simulink library "monroe_library"  (R2012b)
settings: Solver=ode45  StartTime=0.0  StopTime=10.0  RelTol=1e-3
values from neighbouring files (symbols this model uses):
  input_bit_width = ', num2str(input_bit_width))    [fft_direct_draw.m]
undefined symbols (not defined in the file or in its folder): gcbh, xlBlockLoadCallback
libraries: xbsIndex_r4 x1880, monroe_library x159, casper_library x13, xps_library x1
(part 1 of 43)
settings Model: Creator=monroe  LastModifiedBy=root

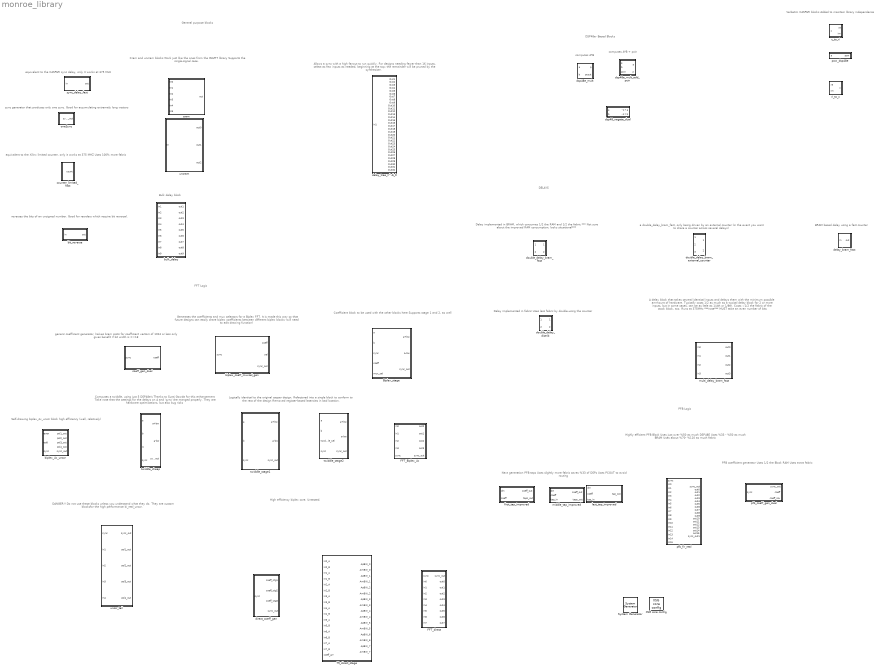
== system monroe_library ==
  note: computes A*B + pcin
  note: equivalent to the CASPER sync delay,
      | only it works at 375 MHz
  note: equivalent to the Xilinx
      | limited counter, only it works at 375 MHZ
      | Uses 100% more fabric
  note: Computes a twiddle, using just 5 DSP48e's
      | Thanks to Suraj Gowda for this enhancement
      | Take note that the settings for the delays on A and 'sync' are manged properly.
      | They are hardware optimizations, but also bug risks
  note: BRAM based delay using a fast counter
  note: sync generator that produces only one sync.
      | Good for accumulating extremely long vectors
  note: computes A*B
  note: Delay implemented in BRAM, which consumes
      | 1/2 the RAM and 1/2 the fabric
      |
      | *** Not sure about the improved RAM consumption; looks situational***
  note: Delay implemented in fabric
      | Uses less fabric by double-using the counter
  note: Next generation PFB taps
      |
      | Uses slightly more fabric
      | saves %33 of DSPs
      | Uses PCOUT to avoid routing
  note: PFB coefficient generator
      | Uses 1/2 the Block RAM
      | Uses extra fabric
  note: Highly efficient PFB Block
      | Uses just over %50 as much DSP48E
      | Uses %33 - %50 as much BRAM
      | Uses about %70- %110 as much fabric
  note: Logically identical to the original casper design.
      | Refactored into a single block to conform to the rest of the design
      | Removed register-based latencies in bad location.
  note: Allows a sync with a high fanout to run quickly.
      |   For designs needing fewer than 16 inputs, select as few inputs as needed, beginning at the top;
      | the remainder will be pruned by the synthesizer.
  note: a double_delay_bram_fast, only being driven by an external counter
      | (in the event you want to share a counter across several delays)
  note: generic coefficient generator,  halves bram costs for coefficient vectors of  1024 or less
      | only gives benefit if bit width is =<18
  note: Cram and uncram blocks
      | Work just like the ones from the GAVRT library
      | Supports the single-signal case.
  note: Generates the coefficients and mux selectors for a Biplex FFT.
      | It is made this way so that future designs can easily share biplex coefficients
      | between different biplex blocks (will need to edit drawing function)
  note: A delay block that takes several identical inputs and
      | delays them with the minimum possible ammount of hardware.
      | Typically costs 1/2 as much as a typical delay block for 2 or more inputs,
      | but in some cases, can be as little as 1/4th or 1/8th.
      | Costs ~1/2 the fabric of the stock block, too.
      | Runs at 375MHz
      |
      | ***note***  MUST take an even number of bits
  note: Verbatim CASPER blocks
      | Added to maintain library independence
  note: DELAYS
  note: PFB Logic
  note: FFT Logic
  note: General purpose blocks
  note: DSP48e- Based Blocks
  note: reverses the bits of an unsigned number.
      | Good for reorders which require bit reversal.
  note: DANGER!!
      | Do not use these blocks unless you understand what they do.
      | They are custom blocksfor the high performance bi_real_unscr.
  note: Coefficient block to be used with the other blocks here
      | Supports stage 1 and 2, as well
  note: Self-drawing biplex_4x_unscr block
      | high efficiency (well, relatively)
  note: High efficiency biplex core.
      | Untested.
  note: Bulk delay block
  " System Generator" : xbsIndex_r4/ System Generator  Tag=genX  xilinxfamily=virtex5  part=xc5vsx95t  speed=-1  package=ff1136  synthesis_tool=XST  clock_wrapper=Clock Enables  directory=./spec_2pol_4kw_6tap_pfb/sysgen  proj_type=Project Navigator  Synth_file=XST Defaults  Impl_file=ISE Defaults  testbench=off  simulink_period=1  sysclk_period=2.6667  dcm_input_clock_period=100  incr_netlist=off  trim_vbits=Everywhere in SubSystem  dbl_ovrd=According to Block Masks  core_generation=According to Block Masks  run_coregen=off  deprecated_control=off  eval_field=0  block_type=sysgen
      settings: block_version=11.4
  Biplex_stage : Subsystem  mask{FFTSize=10, FFTStage=3, input_bit_width=18, coeff_bit_width=18, output_bit_width=18, delays_bram=0, bram_latency=2, shift=0, delay_arr=[0,1,0]}
      mask prompts: FFTSize "FFT Size"; FFTStage "FFT Stage"; input_bit_width "Input Bit Width"; coeff_bit_width "Coefficient Bit Width"; output_bit_width "Output Bit Width"; delays_bram "Delays in BRAM"; bram_latency "BRAM latency"; shift "Downshift in this stage? (0 or 1)"; delay_arr "In-Stage Delay Array"
      mask init:
      | config.source=str2func('biplex_stage_n_draw');
      | config.toplevel=gcb;
      | config.debug=0;
      | config.depend={'biplex_stage_n_draw.m'};
      | xBlock(config,{FFTSize, FFTStage, input_bit_width, coeff_bit_width, output_bit_width, delays_bram, bram_latency, shift, delay_arr});
  FFT_Biplex_4x : Subsystem  mask{FFTSize=10, coeff_bit_width=18, input_bit_width=18, output_bit_width=18, inter_stage_bit_width=18, shift_arr=1, mux_latency_arr=0, max_distro_size_coeff=4, max_distro_size_delay=3, register_coeffs=off, stage_pre_delay=off, stage_mid_delay=off, stage_post_delay=off, bram_latency_fft=off, bram_latency_unscr=off, unscr_din_latency=off}
      mask prompts: FFTSize "FFT Size (2^?) points"; coeff_bit_width "Coefficient Bit Width"; input_bit_width "Input Bit Width"; output_bit_width "Output Bit Width"; inter_stage_bit_width "Inter-Stage Bit Widths"; shift_arr "Shift after n-th stage? (array of FFTSize elements, each a 0 or 1)"; mux_latency_arr "Mux Latency Array"; max_distro_size_coeff "When to start putting Coefficients in BRAM (after 2^? elements)"; max_distro_size_delay "When to start putting Delays in BRAM (after 2^? latency)"; register_coeffs "Register Coefficients?"; stage_pre_delay "Stage Pre-delay? (0 or 1)"; stage_mid_delay "Stage Mid-Delay? (0 or 1)"; stage_post_delay "Stage Post-Delay? (0 or 1)"; bram_latency_fft "Register Bram outputs? (FFT)"; bram_latency_unscr "Register Bram outputs? (Unscrambler)"; unscr_din_latency "Register Unscrambler Reorder inputs?"
      mask init:
      | config.source=str2func('fft_biplex_4x_draw');
      | config.toplevel=gcb;
      | config.debug=0;
      | config.depend={'fft_biplex_4x_draw.m'};
      | xBlock(config,{FFTSize,coeff_bit_width,input_bit_width,output_bit_width,inter_stage_bit_width,shift_arr,max_distro_size_coeff,max_distro_size_delay,register_coeffs,stage_pre_delay,stage_mid_delay,stage_post_delay,mux_latency_arr,bram_latency_fft+2,bram_latency_unscr+2,unscr_din_latency});
  FFT_direct : Subsystem  mask{FFTSize=3, larger_fft_size=9, input_bit_width=18, coeff_bit_width=18, inter_stage_bit_width=18, output_bit_width=18, register_coeffs=on, delay_input=on, delay_output=off, sync_tree_input=off, optional_delay_arr=1, coeff_group_arr_in=[], coeff_stage_step_arr=0, shift_arr=1}
      mask prompts: FFTSize "FFT Size"; larger_fft_size "Larger FFT Size"; input_bit_width "Input Bit Width (no more than 24)"; coeff_bit_width "Coeff Bit Width (Array, FFT Size long; max 18)"; inter_stage_bit_width "Inter-Stage Bit Width (Array, FFT Size -1 long, max 24)"; output_bit_width "Output Bit Width (positive integer)"; register_coeffs "Register Coefficients?"; delay_input "Delay Input?"; delay_output "Delay Output?"; sync_tree_input "Add Sync Tree to Input?"; optional_delay_arr "Optional Delays (array, FFT Size-1 long)"; coeff_group_arr_in "Coefficient Grouping Array (read documentation or use empty array  []   )"; coeff_stage_step_arr "Coefficient Stage Step Size (array of FFT Size, non-negative integers)"; shift_arr "Stage Shift Array (array of FFT Size, non-negative integers; recomend ones(1,FFTSize))"
      mask init:
      | config.source=str2func('fft_direct_draw');
      | config.toplevel=gcb;
      | config.debug=0;
      | config.depend={'fft_direct_draw.m'};
      | xBlock(config,{FFTSize,larger_fft_size,input_bit_width,coeff_bit_width,inter_stage_bit_width,output_bit_width,register_coeffs,delay_input,delay_output,sync_tree_input,optional_delay_arr,coeff_group_arr_in,coeff_stage_step_arr,shift_arr});
  XSG core config : xps_library/XSG core config  Tag=xps:xsg  hw_sys=ROACH:sx95t  clk_src=adc0_clk  ROACH_clk_src=adc0_clk  ROACH2_clk_src=adc0_clk  clk_rate=375  sample_period=1  synthesis_tool=XST
  biplex_4x_unscr : Subsystem  mask{FFTSize=9, bram_latency=3, input_bit_width=18, reorder_din_latency=1}
      mask prompts: FFTSize "Size of FFT (2^?):"; bram_latency "BRAM Latency"; input_bit_width "Input Bit Width"; reorder_din_latency "Reorder Data In Latency"
      mask init:
      | config.source=str2func('biplex_4x_unscr_draw');
      | config.toplevel=gcb;
      | config.debug=0;
      | config.depend={'biplex_4x_unscr_draw.m'};
      | xBlock(config,{FFTSize, bram_latency, input_bit_width, reorder_din_latency});
  biplex_coeff_muxsel_gen : Subsystem  mask{FFTSize=4, bit_width=18*ones(1,2), register_coeffs=0, max_distro_size=4, optional_delay_arr=[[1,1,1]; [1,1,1];  [1,1,1];  [1,1,1]], stage_delay_arr=[3,6,6,6]}
      mask prompts: FFTSize "FFT Size"; bit_width "Coefficient Bit Width"; register_coeffs "Register Coeffs?"; max_distro_size "Maximum number of coeffs to put in distributed memory? (2^? points)"; optional_delay_arr "In-Stage Delay Array"; stage_delay_arr "Mandatory Stage Delay Array"
      mask init:
      | config.source=str2func('biplex_coeff_muxsel_gen_draw');
      | config.toplevel=gcb;
      | config.debug=0;
      | config.depend={'biplex_coeff_muxsel_gen_draw.m'};
      | xBlock(config,{FFTSize, bit_width, register_coeffs, max_distro_size, optional_delay_arr, stage_delay_arr});
  bit_reverse : Subsystem  mask{nBits=5}
      mask prompts: nBits "# bits?"
      mask init:
      | config.source=str2func('bit_reverse_draw');
      | config.toplevel=gcb;
      | config.debug=0;
      | config.depend={'bit_reverse_draw.m'};
      | xBlock(config,{nBits,1});
  bulk_delay : Subsystem  mask{numInputs=9, delay_arr=5}
      mask prompts: numInputs "# Inputs?"; delay_arr "Delays (integer or array of #inputs elements)"
      mask init:
      | config.source=str2func('bulk_delay_draw');
      | config.toplevel=gcb;
      | config.debug=0;
      | config.depend={'bulk_delay_draw.m'};
      | xBlock(config,{numInputs,delay_arr});
  c_to_ri : Subsystem  AncestorBlock=casper_library/Misc/c_to_ri  mask(c_to_ri){n_bits=8, bin_pt=7}
      mask prompts: n_bits "Bit Width"; bin_pt "Binary Point"
      mask help:
      | Outputs real and imaginary components of a complex input.
      | Useful for simplifying interconnects.
      | See also: Real-Imag to Complex (ri_to_c)
      mask init:
      | annotation=sprintf('%d_%d r/i',n_bits,bin_pt);
      | set_param(gcb,'AttributesFormatString',annotation);
      settings: AttributesFormatString=8_7 r/i
      mask Help: eval('xlWeb(''http://casper.berkeley.edu/wiki/C_to_ri'')')
  coeff_gen_dual : Subsystem  mask{coeff=(1:128)/128, memory_type=Block RAM, bit_width=18, register_output=0, step_rate=0}
      mask prompts: coeff "Coefficients"; memory_type "Memory Type"; bit_width "Bit Width"; register_output "Register Output? (does not affect latency)"; step_rate "Step Rate"
      mask init:
      | config.source=str2func('coeff_gen_dual_draw');
      | config.toplevel=gcb;
      | config.debug=0;
      | config.depend={'coeff_gen_dual_draw.m'};
      | xBlock(config,{coeff, memory_type, bit_width, step_rate, register_output});
      mask TypeOptions memory_type: Block RAM | Distributed memory
  counter_limited_fast : Subsystem  mask{bit_width=8, count_to=250, register_output=0, cheap_counter=0}
      mask prompts: bit_width "Bit Width"; count_to "Max Counter Value"; register_output "Register Output? (0 or 1)"; cheap_counter "Use Cheap Counter Instead?"
  cram : Subsystem  mask{numInputs=6}
      mask prompts: numInputs "# Inputs"
      mask init:
      | config.source=str2func('cram_draw');
      | config.toplevel=gcb;
      | config.debug=0;
      | config.depend={'cram_draw.m'};
      | xBlock(config,{numInputs});
  delay_bram_fast : Subsystem  AncestorBlock=monroe_library/tap1/delay_bram  mask{delay_len=1024, bram_latency=2, memory_type=Block RAM, register_counter=0}
      mask prompts: delay_len "Delay Length"; bram_latency "Bram Latency"; memory_type "Memory Type"; register_counter "Register internal counter? (0 or 1)"
      mask TypeOptions memory_type: Block RAM | Distributed Memory
  delay_tree_z^-6_0 : Subsystem
  direct_coeff_gen : Subsystem  mask{fft_size=3, larger_fft_size=13, bit_width=18*ones(1,3), register_coeffs=0, delay_input=1, sync_tree_input=0, optional_delay_arr=[1,1,1], coeff_group_arr=[], coeff_stage_step_arr=zeros(1,3)}
      mask prompts: fft_size "FFT Size"; larger_fft_size "Larger FFT Size"; bit_width "Coeff bit width"; register_coeffs "Register Coefficients"; delay_input "Register Inputs"; sync_tree_input "Attach Sync-Tree to input (0 or 1)"; optional_delay_arr "Optional Delay Array"; coeff_group_arr "Coeff Group Array"; coeff_stage_step_arr "Coeff Stage Step Array"
      mask init:
      | config.source=str2func('direct_coeff_gen_draw');
      | config.toplevel=gcb;
      | config.debug=0;
      | config.depend={'direct_coeff_gen_draw.m'};
      | xBlock(config,{fft_size, larger_fft_size, bit_width, register_coeffs, delay_input, sync_tree_input, optional_delay_arr, coeff_group_arr, coeff_stage_step_arr});
  double_delay_bram_external_counter : Subsystem  mask{delay_len=1024, bram_latency=2}
      mask prompts: delay_len "Delay Length"; bram_latency "Bram Latency"
  double_delay_bram_fast : Subsystem  mask{delay_len=1024, bram_latency=2, register_counter=0}
      mask prompts: delay_len "Delay Length"; bram_latency "Bram Latency"; register_counter "Register Internal Counter? (0 or 1)"
  double_delay_distrib : Subsystem  mask{delay_len=1024, bram_latency=2}
      mask prompts: delay_len "Delay Length"; bram_latency "Bram Latency"
  dsp48_negate_dual : Subsystem  mask{a_bit_width=input_bit_width, a_bin_pt=input_bit_width-1}
      mask prompts: a_bit_width "bit width"; a_bin_pt "binary point"
  dsp48e_mult : Subsystem  mask{a_bin_pt=17, b_bin_pt=17}
      mask prompts: a_bin_pt "'A' binal point"; b_bin_pt "'B' binal point"
  dsp48e_mult_add_pcin : Subsystem  mask{a_bin_pt=0, b_bin_pt=0}
      mask prompts: a_bin_pt "'A' binal point"; b_bin_pt "'B' binal point"
  fft_direct_stage : Subsystem  mask{FFTSize=4, FFTStage=3, input_bit_width=18, coeff_bit_width=18, output_bit_width=18, shift=1}
      mask prompts: FFTSize "FFT Size"; FFTStage "FFT Stage"; input_bit_width "Input Bit Width"; coeff_bit_width "Coeff Bit Width"; output_bit_width "Output Bit Width"; shift "Downshift stage output?"
      mask init:
      | config.source=str2func('fft_direct_stage_draw');
      | config.toplevel=gcb;
      | config.debug=0;
      | config.depend={'fft_direct_stage_draw.m'};
      | xBlock(config,{FFTSize, FFTStage, input_bit_width, coeff_bit_width, output_bit_width, shift});
  first_tap_improved : Subsystem  AncestorBlock=casper_library/PFBs/tap_real  mask{data_bin_pt=17, coeff_bit_width=18}
      mask prompts: data_bin_pt "Data Binal Point"; coeff_bit_width "Coefficient Bit Width (max 25)"
  last_tap_improved : Subsystem  AncestorBlock=casper_library/PFBs/last_tap_real  mask{data_bin_pt=17, coeff_bin_pt=17, stage_num=6}
      mask prompts: data_bin_pt "Data Binal Point"; coeff_bin_pt "Coeficient Binal Point"; stage_num "Stage Number"
  middle_tap_improved : Subsystem  mask{data_bin_pt=17, coeff_bit_width=18, stage_num=2}
      mask prompts: data_bin_pt "Data Binal Point"; coeff_bit_width "Coefficient Bit Width (max 25)"; stage_num "Stage Number"
  multi_delay_bram_fast : Subsystem  mask{numSignals=4, delay_len=1024, bitWidth=18, binPt=17, signalType=Signed, bram_latency=2, register_counter=0}
      mask prompts: numSignals "# signals"; delay_len "Delay Length"; bitWidth "Bit Width"; binPt "Binal Point"; signalType "Signal Type"; bram_latency "Bram Latency"; register_counter "Register internal counter? (0 or 1)"
      mask init:
      | config.source=str2func('multi_delay_bram_fast_draw');
      | config.toplevel=gcb;
      | config.debug=0;
      | config.depend={'multi_delay_bram_fast_draw.m','cram_draw.m', 'uncram_draw.m'};
      | xBlock(config,{numSignals, delay_len, bitWidth, binPt, signalType, bram_latency,register_counter});
      mask TypeOptions signalType: Signed | Unsigned
  oneSync : Subsystem
  pfb_coeff_gen_dual : Subsystem  mask(pfb_coeff_gen_dual){pfb_size=14, n_sim_inputs=4, n_taps=4, input_num=4, n_bits=18, window_fn=hamming, mem_type=Block RAM, bram_latency=3, bin_width=1}
      mask prompts: pfb_size "PFB Size (2^?)"; n_sim_inputs "# Simultaneous Inputs (2^?)"; n_taps "# Taps"; input_num "Input Number (zero-indexed)"; n_bits "# Coefficient Bits"; window_fn "Window Function"; mem_type "Memory Type"; bram_latency "Bram Latency (reccomend 3)"; bin_width "Channel Width"
      mask init:
      | % wampum=55;
      | % 
      | config.source = str2func('pfb_coeff_gen_dual_draw');
      | config.toplevel=gcb;
      | config.debug=0;
      | config.depend = {'pfb_coeff_gen_dual_draw.m'};
      | 
      | %parameters to pass to drawer
      |     global drawing_parameters;
      |     drawing_parameters.pfb_size=pfb_size;
      |     drawing_parameters.n_sim_inputs=n_sim_inputs;
      |     drawing_parameters.n_taps=n_taps;
      |     drawing_parameters.input_num=input_num;
      |     drawing_parameters.n_bits=n_bits;
      |     drawing_parameters.window_fn=window_fn;
      |     drawing_parameters.mem_type=mem_type;
      |     drawing_parameters.bram_latency=bram_latency;
      |     drawing_parameters.bin_width=bin_width;
      |     drawing_parameters.params_from_struct = 0;
      |     
      | 
      | 
      | xBlock(config, {pfb_size,n_sim_inputs,n_taps,input_num,n_bits,window_fn,mem_type,bram_latency,bin_width})
      | 
      | % %pfb_coeff_gen_dual_draw('pfb_size', pfb_size,'n_sim_inputs',n_sim_inputs,'n_taps',n_taps,'input_num',input_num,'n_bits',n_bits,'window_fn',window_fn,'mem_type',mem_type,'bram_latency',bram_latency,'bin_width',bin_width)
      mask TypeOptions window_fn: bartlett | barthannwin | blackman | blackmanharris | bohamwin | chebwin | flattopwin | gausswin | hamming | hann | kaiser | nuttallwin | parzenwin | rectwin | tukeywin | triang
      mask TypeOptions mem_type: Block RAM | Distributed Memory
  pfb_fir_real : Subsystem  mask(pfb_coeff_gen_dual){pfb_size=14, n_sim_inputs=4, n_taps=4, data_n_bits=18, coeff_n_bits=18, output_bit_width=18, window_fn=hamming, bin_width=1, end_scale_val=1, endDelay=off, cheap_sync=off, autoplace_mode='Attached to both ADC0 and ADC1 (interleaved)', autoplace_optimize=off, bram_latency_coeff=off, bram_latency_delay=off, register_counter=off, pack_delays=on}
      mask prompts: pfb_size "PFB Size (2^?)"; n_sim_inputs "# Simultaneous Inputs (2^?); Max=6"; n_taps "# Taps"; data_n_bits "Input bit Width"; coeff_n_bits "# Coefficient Bits"; output_bit_width "Output bit width"; window_fn "Window Function"; bin_width "Channel Width"; end_scale_val "Downscale at end (2^?)"; endDelay "Delay at end?"; cheap_sync "Use cheap Sync hardware?"; autoplace_mode "Autoplacement Mode?"; autoplace_optimize "Optimize parameters for auto-placement? (settings below here ignored)"; bram_latency_coeff "Regoster Coefficient Brams?"; bram_latency_delay "Register Delay Brams?"; register_counter "Register Delay Counters? (0 or 1)"; pack_delays "Pack delays cross-input?"
      mask init:
      | global drawing_parameters;
      | % drawing_parameters.pfb_size=pfb_size;
      | % drawing_parameters.n_sim_inputs=n_sim_inputs;
      | % drawing_parameters.n_taps=n_taps;
      | % drawing_parameters.data_n_bits=data_n_bits;
      | % drawing_parameters.data_bin_pt=data_bin_pt;
      | % drawing_parameters.coeff_n_bits=coeff_n_bits;
      | % drawing_parameters.coeff_bin_pt=coeff_n_bits-1;
      | % drawing_parameters.window_fn=window_fn;
      | % drawing_parameters.mem_type=mem_type;
      | % drawing_parameters.bram_latency=bram_latency;
      | % drawing_parameters.bin_width=bin_width;
      | % drawing_parameters.end_scale_val=end_scale_val;
      | % drawing_parameters.cheap_sync=cheap_sync;
      | config.source=str2func('pfb_improved_draw');
      | config.toplevel=gcb;
      | config.debug=0;
      | config.depend={'pfb_improved_draw.m','pfb_coeff_gen_dual_draw.m'};
      | xBlock(config,{pfb_size,n_sim_inputs,n_taps,data_n_bits,coeff_n_bits, ...
      |                output_bit_width,window_fn,bram_latency_coeff+2,bram_latency_delay+2,bin_width,end_scale_val,endDelay, cheap_sync,register_counter, pack_delays, autoplace_mode, autoplace_optimize});
      mask TypeOptions window_fn: bartlett | barthannwin | blackman | blackmanharris | bohamwin | chebwin | flattopwin | gausswin | hamming | hann | kaiser | nuttallwin | parzenwin | rectwin | tukeywin | triang
      mask TypeOptions autoplace_mode: 'Attached to ADC0' | 'Attached to ADC1' | 'Attached to both ADC0 and ADC1 (interleaved)'
  pow_dsp48e : Subsystem  AncestorBlock=casper_library/Misc/pow_dsp48e  mask{bit_width=8}
      mask prompts: bit_width "Bit Width"
  ri_to_c : Subsystem  AncestorBlock=casper_library/Misc/ri_to_c  mask(ri_to_c){}
      mask help:
      | Concatenates real and imaginary inputs into a complex output.
      | Useful for simplifying interconnects.
      | See also: Complex to Real-Imag (c_to_ri)
      mask Help: eval('xlWeb(''http://casper.berkeley.edu/wiki/Ri_to_c'')')
  sync_delay_fast : Subsystem  mask{delay_len=1024}
      mask prompts: delay_len "Delay Length"
      mask Display: fprintf('Z^-%d', delay_len)
  twiddle_cheap : Subsystem  AncestorBlock=monroe_library/twiddle_cheap  mask{a_n_bits=18, a_bin_pt=17, b_n_bits=18, b_bin_pt=17, w_n_bits=18, w_bin_pt=17, a_delay=0, apbw_delay=0, out_n_bits=18, downshift_at_end=0}
      mask prompts: a_n_bits "# bits A"; a_bin_pt "A binal point"; b_n_bits "# bits B"; b_bin_pt "B binal point"; w_n_bits "# bits W"; w_bin_pt "W binal point"; a_delay "Delay 'A' in-block? (0 or 1)"; apbw_delay "Delay 'A+BW' in-block? (0 or 1)"; out_n_bits "#bits Out"; downshift_at_end "Downshift at end? (0 or 1)"
  twiddle_stage1 : Subsystem  AncestorBlock=monroe_library/twiddle_stage1  mask(twiddle_pass_through){input_bit_width=18, out_n_bits=0, downshift_at_end=0}
      mask prompts: input_bit_width "Input Bit Width"; out_n_bits "Output Bit Width"; downshift_at_end "Downshift at end"
      mask help:
      | Used in FFT library. Used when coefficients
      | are 2^0 i.e just pass data through without delays
  twiddle_stage2 : Subsystem  AncestorBlock=casper_library/FFTs/Twiddle/twiddle_pass_through  mask(twiddle_pass_through){FFTSize=10, input_bit_width=18, out_n_bits=0, downshift_at_end=0}
      mask prompts: FFTSize "FFT Size"; input_bit_width "Input Bit Width"; out_n_bits "Output  Bit Width"; downshift_at_end "Downshift at end (0 or 1)"
      mask help:
      | Used in FFT library. Used when coefficients
      | are 2^0 i.e just pass data through without delays
  uncram : Subsystem  mask{numInputs=3, bitWidth=18, binPt=17, signalType=Signed}
      mask prompts: numInputs "# Inputs"; bitWidth "Bit Width"; binPt "Binal Point"; signalType "Signal Type"
      mask init:
      | config.source=str2func('uncram_draw');
      | config.toplevel=gcb;
      | config.debug=0;
      | config.depend={'uncram_draw.m'};
      | xBlock(config,{numInputs,bitWidth,binPt,signalType});
      mask TypeOptions signalType: Signed | Unsigned
  unscr_tail : Subsystem  AncestorBlock=monroe_library/unscr_tail  mask{FFTSize=5, input_bit_width=18, bram_latency=2, reorder_din_latency=0}
      mask prompts: FFTSize "FFT Size"; input_bit_width "Input Bit Width"; bram_latency "BRAM Latency"; reorder_din_latency "Reorder DIN Latency"

== system monroe_library/Biplex_stage ==
  a : Inport
  b : Inport  Port=2
  sync : Inport  Port=3
  coeff : Inport  Port=4
  mux_sel : Inport  Port=5
  Mux : xbsIndex_r4/Mux  inputs=2  en=off  latency=0  precision=Full  arith_type="Signed  (2's comp)"  n_bits=8  bin_pt=2  quantization=Truncate  overflow=Wrap  dbl_ovrd=off  block_type=mux
  Mux1 : xbsIndex_r4/Mux  inputs=2  en=off  latency=0  precision=Full  arith_type="Signed  (2's comp)"  n_bits=8  bin_pt=2  quantization=Truncate  overflow=Wrap  dbl_ovrd=off  block_type=mux
  delay_ddbf_1 : xbsIndex_r4/Delay  en=off  latency=128  dbl_ovrd=off  reg_retiming=off  block_type=delay
  delay_ddbf_2 : xbsIndex_r4/Delay  en=off  latency=128  dbl_ovrd=off  reg_retiming=off  block_type=delay
  delay_end : xbsIndex_r4/Delay  en=off  latency=2  dbl_ovrd=off  reg_retiming=off  block_type=delay
  delay_mid : xbsIndex_r4/Delay  en=off  latency=2  dbl_ovrd=off  reg_retiming=off  block_type=delay
  delay_mid1 : xbsIndex_r4/Delay  en=off  latency=1  dbl_ovrd=off  reg_retiming=off  block_type=delay
  sync_delay_fast : monroe_library/sync_delay_fast  SystemSampleTime=-1  delay_len=128
  twiddle_cheap : monroe_library/twiddle_cheap  SystemSampleTime=-1  a_n_bits=18  a_bin_pt=17  b_n_bits=18  b_bin_pt=17  w_n_bits=18  w_bin_pt=17  a_delay=0  apbw_delay=0  out_n_bits=18  downshift_at_end=0
  a+bw : Outport
  a-bw : Outport  Port=2
  sync_out : Outport  Port=3
  wires:
  mux_sel/1 -> Mux1/1, Mux/1
  delay_ddbf_2/1 -> Mux1/3, Mux/2
  a/1 -> Mux1/2, Mux/3
  twiddle_cheap/3 -> sync_out/1
  twiddle_cheap/2 -> a-bw/1
  twiddle_cheap/1 -> delay_end/1
  sync_delay_fast/1 -> twiddle_cheap/4
  coeff/1 -> twiddle_cheap/3
  delay_mid1/1 -> twiddle_cheap/2
  delay_mid/1 -> twiddle_cheap/1
  sync/1 -> sync_delay_fast/1
  b/1 -> delay_ddbf_2/1
  Mux/1 -> delay_mid1/1
  delay_ddbf_1/1 -> delay_mid/1
  delay_end/1 -> a+bw/1
  Mux1/1 -> delay_ddbf_1/1

== system monroe_library/FFT_Biplex_4x ==
  in0 : Inport
  in1 : Inport  Port=2
  in2 : Inport  Port=3
  in3 : Inport  Port=4
  sync : Inport  Port=5
  biplex_4x_unscr : Subsystem
  biplex_muxsel_gen : Subsystem
  coeff_slice10 : xbsIndex_r4/Slice  nbits=36  boolean_output=off  mode=Upper Bit Location + Width  bit1=-252  base1=MSB of Input  bit0=-252  base0=MSB of Input  dbl_ovrd=off  block_type=slice
  coeff_slice3 : xbsIndex_r4/Slice  nbits=36  boolean_output=off  mode=Upper Bit Location + Width  bit1=-0  base1=MSB of Input  bit0=-0  base0=MSB of Input  dbl_ovrd=off  block_type=slice
  coeff_slice4 : xbsIndex_r4/Slice  nbits=36  boolean_output=off  mode=Upper Bit Location + Width  bit1=-36  base1=MSB of Input  bit0=-36  base0=MSB of Input  dbl_ovrd=off  block_type=slice
  coeff_slice5 : xbsIndex_r4/Slice  nbits=36  boolean_output=off  mode=Upper Bit Location + Width  bit1=-72  base1=MSB of Input  bit0=-72  base0=MSB of Input  dbl_ovrd=off  block_type=slice
  coeff_slice6 : xbsIndex_r4/Slice  nbits=36  boolean_output=off  mode=Upper Bit Location + Width  bit1=-108  base1=MSB of Input  bit0=-108  base0=MSB of Input  dbl_ovrd=off  block_type=slice
  coeff_slice7 : xbsIndex_r4/Slice  nbits=36  boolean_output=off  mode=Upper Bit Location + Width  bit1=-144  base1=MSB of Input  bit0=-144  base0=MSB of Input  dbl_ovrd=off  block_type=slice
  coeff_slice8 : xbsIndex_r4/Slice  nbits=36  boolean_output=off  mode=Upper Bit Location + Width  bit1=-180  base1=MSB of Input  bit0=-180  base0=MSB of Input  dbl_ovrd=off  block_type=slice
  coeff_slice9 : xbsIndex_r4/Slice  nbits=36  boolean_output=off  mode=Upper Bit Location + Width  bit1=-216  base1=MSB of Input  bit0=-216  base0=MSB of Input  dbl_ovrd=off  block_type=slice
  cram0 : Subsystem
  cram1 : Subsystem
  sel_slice1 : xbsIndex_r4/Slice  nbits=1  boolean_output=on  mode=Upper Bit Location + Width  bit1=-0  base1=MSB of Input  bit0=-0  base0=MSB of Input  dbl_ovrd=off  block_type=slice
  sel_slice10 : xbsIndex_r4/Slice  nbits=1  boolean_output=on  mode=Upper Bit Location + Width  bit1=-9  base1=MSB of Input  bit0=-9  base0=MSB of Input  dbl_ovrd=off  block_type=slice
  sel_slice2 : xbsIndex_r4/Slice  nbits=1  boolean_output=on  mode=Upper Bit Location + Width  bit1=-1  base1=MSB of Input  bit0=-1  base0=MSB of Input  dbl_ovrd=off  block_type=slice
  sel_slice3 : xbsIndex_r4/Slice  nbits=1  boolean_output=on  mode=Upper Bit Location + Width  bit1=-2  base1=MSB of Input  bit0=-2  base0=MSB of Input  dbl_ovrd=off  block_type=slice
  sel_slice4 : xbsIndex_r4/Slice  nbits=1  boolean_output=on  mode=Upper Bit Location + Width  bit1=-3  base1=MSB of Input  bit0=-3  base0=MSB of Input  dbl_ovrd=off  block_type=slice
  sel_slice5 : xbsIndex_r4/Slice  nbits=1  boolean_output=on  mode=Upper Bit Location + Width  bit1=-4  base1=MSB of Input  bit0=-4  base0=MSB of Input  dbl_ovrd=off  block_type=slice
  sel_slice6 : xbsIndex_r4/Slice  nbits=1  boolean_output=on  mode=Upper Bit Location + Width  bit1=-5  base1=MSB of Input  bit0=-5  base0=MSB of Input  dbl_ovrd=off  block_type=slice
  sel_slice7 : xbsIndex_r4/Slice  nbits=1  boolean_output=on  mode=Upper Bit Location + Width  bit1=-6  base1=MSB of Input  bit0=-6  base0=MSB of Input  dbl_ovrd=off  block_type=slice
  sel_slice8 : xbsIndex_r4/Slice  nbits=1  boolean_output=on  mode=Upper Bit Location + Width  bit1=-7  base1=MSB of Input  bit0=-7  base0=MSB of Input  dbl_ovrd=off  block_type=slice
  sel_slice9 : xbsIndex_r4/Slice  nbits=1  boolean_output=on  mode=Upper Bit Location + Width  bit1=-8  base1=MSB of Input  bit0=-8  base0=MSB of Input  dbl_ovrd=off  block_type=slice
  stage_1 : Subsystem
  stage_10 : Subsystem
  stage_2 : Subsystem
  stage_3 : Subsystem
  stage_4 : Subsystem
  stage_5 : Subsystem
  stage_6 : Subsystem
  stage_7 : Subsystem
  stage_8 : Subsystem
  stage_9 : Subsystem
  out0 : Outport
  out1 : Outport  Port=2
  out2 : Outport  Port=3
  out3 : Outport  Port=4
  sync_out : Outport  Port=5
  wires:
  sync/1 -> stage_1/3(sync), biplex_muxsel_gen/1(sync)
  biplex_muxsel_gen/2(sel) -> sel_slice10/1, sel_slice9/1, sel_slice8/1, sel_slice7/1, sel_slice6/1, sel_slice5/1, sel_slice4/1, sel_slice3/1, sel_slice2/1, sel_slice1/1
  biplex_muxsel_gen/1(coeff) -> coeff_slice10/1, coeff_slice9/1, coeff_slice8/1, coeff_slice7/1, coeff_slice6/1, coeff_slice5/1, coeff_slice4/1, coeff_slice3/1
  biplex_4x_unscr/5(sync_out) -> sync_out/1
  biplex_4x_unscr/4(pol4_out) -> out3/1
  biplex_4x_unscr/3(pol3_out) -> out2/1
  biplex_4x_unscr/2(pol2_out) -> out1/1
  biplex_4x_unscr/1(pol1_out) -> out0/1
  biplex_muxsel_gen/3(sync_out) -> biplex_4x_unscr/3(sync)
  stage_10/2(a-bw) -> biplex_4x_unscr/2(odd)
  stage_10/1(a+bw) -> biplex_4x_unscr/1(even)
  sel_slice10/1 -> stage_10/5(mux_sel)
  coeff_slice10/1 -> stage_10/4(coeff)
  stage_9/3(sync_out) -> stage_10/3(sync)
  stage_9/2(a-bw) -> stage_10/2(b)
  stage_9/1(a+bw) -> stage_10/1(a)
  sel_slice9/1 -> stage_9/5(mux_sel)
  coeff_slice9/1 -> stage_9/4(coeff)
  stage_8/3(sync_out) -> stage_9/3(sync)
  stage_8/2(a-bw) -> stage_9/2(b)
  stage_8/1(a+bw) -> stage_9/1(a)
  sel_slice8/1 -> stage_8/5(mux_sel)
  coeff_slice8/1 -> stage_8/4(coeff)
  stage_7/3(sync_out) -> stage_8/3(sync)
  stage_7/2(a-bw) -> stage_8/2(b)
  stage_7/1(a+bw) -> stage_8/1(a)
  sel_slice7/1 -> stage_7/5(mux_sel)
  coeff_slice7/1 -> stage_7/4(coeff)
  stage_6/3(sync_out) -> stage_7/3(sync)
  stage_6/2(a-bw) -> stage_7/2(b)
  stage_6/1(a+bw) -> stage_7/1(a)
  sel_slice6/1 -> stage_6/5(mux_sel)
  coeff_slice6/1 -> stage_6/4(coeff)
  stage_5/3(sync_out) -> stage_6/3(sync)
  stage_5/2(a-bw) -> stage_6/2(b)
  stage_5/1(a+bw) -> stage_6/1(a)
  sel_slice5/1 -> stage_5/5(mux_sel)
  coeff_slice5/1 -> stage_5/4(coeff)
  stage_4/3(sync_out) -> stage_5/3(sync)
  stage_4/2(a-bw) -> stage_5/2(b)
  stage_4/1(a+bw) -> stage_5/1(a)
  sel_slice4/1 -> stage_4/5(mux_sel)
  coeff_slice4/1 -> stage_4/4(coeff)
  stage_3/3(sync_out) -> stage_4/3(sync)
  stage_3/2(a-bw) -> stage_4/2(b)
  stage_3/1(a+bw) -> stage_4/1(a)
  sel_slice3/1 -> stage_3/5(mux_sel)
  coeff_slice3/1 -> stage_3/4(coeff)
  stage_2/3(sync_out) -> stage_3/3(sync)
  stage_2/2(a-bw) -> stage_3/2(b)
  stage_2/1(a+bw) -> stage_3/1(a)
  sel_slice2/1 -> stage_2/4(mux_sel)
  stage_1/3(sync_out) -> stage_2/3(sync)
  stage_1/2(a-bw) -> stage_2/2(b)
  stage_1/1(a+bw) -> stage_2/1(a)
  sel_slice1/1 -> stage_1/4(mux_sel)
  cram1/1(out) -> stage_1/2(b)
  cram0/1(out) -> stage_1/1(a)
  in3/1 -> cram1/2(in1)
  in2/1 -> cram1/1(in0)
  in1/1 -> cram0/2(in1)
  in0/1 -> cram0/1(in0)

== system monroe_library/FFT_direct ==
  sync : Inport
  in0 : Inport  Port=2
  in1 : Inport  Port=3
  in2 : Inport  Port=4
  in3 : Inport  Port=5
  in4 : Inport  Port=6
  in5 : Inport  Port=7
  in6 : Inport  Port=8
  in7 : Inport  Port=9
  bulk_delay_0_1 : Subsystem
  bulk_delay_1_1 : Subsystem
  bulk_delay_2_1 : Subsystem
  bulk_delay_3_1 : Subsystem
  direct_coeff_gen : Subsystem
  stage_1 : Subsystem
  stage_2 : Subsystem
  stage_3 : Subsystem
  sync_out : Outport
  out0 : Outport  Port=2
  out1 : Outport  Port=3
  out2 : Outport  Port=4
  out3 : Outport  Port=5
  out4 : Outport  Port=6
  out5 : Outport  Port=7
  out6 : Outport  Port=8
  out7 : Outport  Port=9
  wires:
  bulk_delay_3_1/8(out8) -> out7/1
  bulk_delay_3_1/7(out7) -> out6/1
  bulk_delay_3_1/6(out6) -> out5/1
  bulk_delay_3_1/5(out5) -> out4/1
  bulk_delay_3_1/4(out4) -> out3/1
  bulk_delay_3_1/3(out3) -> out2/1
  bulk_delay_3_1/2(out2) -> out1/1
  bulk_delay_3_1/1(out1) -> out0/1
  stage_3/8(AmBW_3) -> bulk_delay_3_1/8(in8)
  stage_3/4(AmBW_1) -> bulk_delay_3_1/7(in7)
  stage_3/6(AmBW_2) -> bulk_delay_3_1/6(in6)
  stage_3/2(AmBW_0) -> bulk_delay_3_1/5(in5)
  stage_3/7(ApBW_3) -> bulk_delay_3_1/4(in4)
  stage_3/3(ApBW_1) -> bulk_delay_3_1/3(in3)
  stage_3/5(ApBW_2) -> bulk_delay_3_1/2(in2)
  stage_3/1(ApBW_0) -> bulk_delay_3_1/1(in1)
  direct_coeff_gen/3(coeff_stg3) -> stage_3/9(coeff_arr)
  bulk_delay_2_1/8(out8) -> stage_3/8(in3_B)
  bulk_delay_2_1/7(out7) -> stage_3/7(in3_A)
  bulk_delay_2_1/6(out6) -> stage_3/6(in2_B)
  bulk_delay_2_1/5(out5) -> stage_3/5(in2_A)
  bulk_delay_2_1/4(out4) -> stage_3/4(in1_B)
  bulk_delay_2_1/3(out3) -> stage_3/3(in1_A)
  bulk_delay_2_1/2(out2) -> stage_3/2(in0_B)
  bulk_delay_2_1/1(out1) -> stage_3/1(in0_A)
  stage_2/8(AmBW_3) -> bulk_delay_2_1/8(in8)
  stage_2/6(AmBW_2) -> bulk_delay_2_1/7(in7)
  stage_2/7(ApBW_3) -> bulk_delay_2_1/6(in6)
  stage_2/5(ApBW_2) -> bulk_delay_2_1/5(in5)
  stage_2/4(AmBW_1) -> bulk_delay_2_1/4(in4)
  stage_2/2(AmBW_0) -> bulk_delay_2_1/3(in3)
  stage_2/3(ApBW_1) -> bulk_delay_2_1/2(in2)
  stage_2/1(ApBW_0) -> bulk_delay_2_1/1(in1)
  direct_coeff_gen/2(coeff_stg2) -> stage_2/9(coeff_arr)
  bulk_delay_1_1/8(out8) -> stage_2/8(in3_B)
  bulk_delay_1_1/7(out7) -> stage_2/7(in3_A)
  bulk_delay_1_1/6(out6) -> stage_2/6(in2_B)
  bulk_delay_1_1/5(out5) -> stage_2/5(in2_A)
  bulk_delay_1_1/4(out4) -> stage_2/4(in1_B)
  bulk_delay_1_1/3(out3) -> stage_2/3(in1_A)
  bulk_delay_1_1/2(out2) -> stage_2/2(in0_B)
  bulk_delay_1_1/1(out1) -> stage_2/1(in0_A)
  stage_1/8(AmBW_3) -> bulk_delay_1_1/8(in8)
  stage_1/4(AmBW_1) -> bulk_delay_1_1/7(in7)
  stage_1/6(AmBW_2) -> bulk_delay_1_1/6(in6)
  stage_1/2(AmBW_0) -> bulk_delay_1_1/5(in5)
  stage_1/7(ApBW_3) -> bulk_delay_1_1/4(in4)
  stage_1/3(ApBW_1) -> bulk_delay_1_1/3(in3)
  stage_1/5(ApBW_2) -> bulk_delay_1_1/2(in2)
  stage_1/1(ApBW_0) -> bulk_delay_1_1/1(in1)
  direct_coeff_gen/1(coeff_stg1) -> stage_1/9(coeff_arr)
  bulk_delay_0_1/8(out8) -> stage_1/8(in3_B)
  bulk_delay_0_1/7(out7) -> stage_1/7(in3_A)
  bulk_delay_0_1/6(out6) -> stage_1/6(in2_B)
  bulk_delay_0_1/5(out5) -> stage_1/5(in2_A)
  bulk_delay_0_1/4(out4) -> stage_1/4(in1_B)
  bulk_delay_0_1/3(out3) -> stage_1/3(in1_A)
  bulk_delay_0_1/2(out2) -> stage_1/2(in0_B)
  bulk_delay_0_1/1(out1) -> stage_1/1(in0_A)
  direct_coeff_gen/4(sync_out) -> sync_out/1
  sync/1 -> direct_coeff_gen/1(sync)
  in7/1 -> bulk_delay_0_1/8(in8)
  in3/1 -> bulk_delay_0_1/7(in7)
  in6/1 -> bulk_delay_0_1/6(in6)
  in2/1 -> bulk_delay_0_1/5(in5)
  in5/1 -> bulk_delay_0_1/4(in4)
  in1/1 -> bulk_delay_0_1/3(in3)
  in4/1 -> bulk_delay_0_1/2(in2)
  in0/1 -> bulk_delay_0_1/1(in1)

== system monroe_library/biplex_4x_unscr ==
  even : Inport
  odd : Inport  Port=2
  sync : Inport  Port=3
  Constant1 : xbsIndex_r4/Constant  arith_type=Unsigned  const=255  n_bits=9  bin_pt=0  explicit_period=on  period=1  equ=P=C  opselect=C  inp2=PCIN>>17  opr=+  inp1=P  carry=CIN  dbl_ovrd=off  block_type=constant
  Constant2 : xbsIndex_r4/Constant  arith_type=Unsigned  const=511  n_bits=9  bin_pt=0  explicit_period=on  period=1  equ=P=C  opselect=C  inp2=PCIN>>17  opr=+  inp1=P  carry=CIN  dbl_ovrd=off  block_type=constant
  Counter : xbsIndex_r4/Counter  cnt_type=Free Running  cnt_to=Inf  operation=Up  start_count=0  cnt_by_val=1  arith_type=Unsigned  n_bits=9  bin_pt=0  load_pin=off  rst=on  en=off  explicit_period=off  period=1  dbl_ovrd=off  use_behavioral_HDL=off  implementation=Fabric  use_rpm=on  block_type=counter
  Delay : xbsIndex_r4/Delay  en=off  latency=1  dbl_ovrd=off  reg_retiming=off  block_type=delay
  Mux{,1..3} (4 alike) : xbsIndex_r4/Mux  inputs=2  en=off  latency=1  precision=Full  arith_type="Signed  (2's comp)"  n_bits=8  bin_pt=2  quantization=Truncate  overflow=Wrap  dbl_ovrd=off  block_type=mux
  Relational : xbsIndex_r4/Relational  mode=a=b  en=off  latency=1  dbl_ovrd=off  block_type=relational
  Relational1 : xbsIndex_r4/Relational  mode=a=b  en=off  latency=1  dbl_ovrd=off  block_type=relational
  double_delay_bram_fast : monroe_library/double_delay_bram_fast  SystemSampleTime=-1  delay_len=256  bram_latency=3  register_counter=0
  dual_bit_reverse : Subsystem
  unscr_tail : monroe_library/unscr_tail  SystemSampleTime=-1  FFTSize=9  input_bit_width=18  bram_latency=3  reorder_din_latency=1
  pol1_out : Outport
  pol2_out : Outport  Port=2
  pol3_out : Outport  Port=3
  pol4_out : Outport  Port=4
  sync_out : Outport  Port=5
  wires:
  Delay/1 -> Mux3/3, Mux2/2, Mux1/3, Mux/2
  Counter/1 -> Relational1/2, Relational/1
  Relational/1 -> Mux3/1, Mux/1
  Relational1/1 -> Mux2/1, Mux1/1
  dual_bit_reverse/1(sync_out) -> unscr_tail/1, Counter/1
  dual_bit_reverse/2(dout0) -> Mux3/2, Mux2/3, Mux1/2, Mux/3
  unscr_tail/5 -> pol4_out/1
  unscr_tail/4 -> pol3_out/1
  unscr_tail/3 -> pol2_out/1
  unscr_tail/2 -> pol1_out/1
  unscr_tail/1 -> sync_out/1
  Mux2/1 -> unscr_tail/5
  Mux3/1 -> unscr_tail/4
  double_delay_bram_fast/2 -> unscr_tail/3
  double_delay_bram_fast/1 -> unscr_tail/2
  dual_bit_reverse/3(dout1) -> Delay/1
  odd/1 -> dual_bit_reverse/3(din1)
  even/1 -> dual_bit_reverse/2(din0)
  sync/1 -> dual_bit_reverse/1(sync)
  Mux/1 -> double_delay_bram_fast/2  "xlsub2_Mux_out1"
  Mux1/1 -> double_delay_bram_fast/1
  Constant1/1 -> Relational1/1
  Constant2/1 -> Relational/2

== system monroe_library/biplex_coeff_muxsel_gen ==
  sync : Inport
  Counter : xbsIndex_r4/Counter  cnt_type=Free Running  cnt_to=Inf  operation=Up  start_count=0  cnt_by_val=1  arith_type=Unsigned  n_bits=4  bin_pt=0  load_pin=off  rst=on  en=off  explicit_period=on  period=1  dbl_ovrd=off  use_behavioral_HDL=off  implementation=Fabric  block_type=counter
  coeff_gen3 : Subsystem
  coeff_gen4 : Subsystem
  coeff_sync_early_3 : xbsIndex_r4/Delay  en=off  latency=17  dbl_ovrd=off  reg_retiming=off  block_type=delay
  coeff_sync_early_4 : xbsIndex_r4/Delay  en=off  latency=9  dbl_ovrd=off  reg_retiming=off  block_type=delay
  coeff_sync_late_3 : xbsIndex_r4/Delay  en=off  latency=2  dbl_ovrd=off  reg_retiming=off  block_type=delay
  coeff_sync_late_4 : xbsIndex_r4/Delay  en=off  latency=1  dbl_ovrd=off  reg_retiming=off  block_type=delay
  concat : xbsIndex_r4/Concat  num_inputs=4  dbl_ovrd=off  block_type=concat
  cram : Subsystem
  delay_sync_final : xbsIndex_r4/Delay  en=off  latency=7  dbl_ovrd=off  reg_retiming=off  block_type=delay
  sel_delay1 : xbsIndex_r4/Delay  en=off  latency=1  dbl_ovrd=off  reg_retiming=off  block_type=delay
  sel_delay2 : xbsIndex_r4/Delay  en=off  latency=6  dbl_ovrd=off  reg_retiming=off  block_type=delay
  sel_delay3 : xbsIndex_r4/Delay  en=off  latency=9  dbl_ovrd=off  reg_retiming=off  block_type=delay
  sel_delay4 : xbsIndex_r4/Delay  en=off  latency=9  dbl_ovrd=off  reg_retiming=off  block_type=delay
  slice_sel_bottom_1 : xbsIndex_r4/Slice  nbits=3  boolean_output=off  mode=Lower Bit Location + Width  bit1=0  base1=LSB of Input  bit0=0  base0=LSB of Input  dbl_ovrd=off  block_type=slice
  slice_sel_bottom_2 : xbsIndex_r4/Slice  nbits=2  boolean_output=off  mode=Lower Bit Location + Width  bit1=0  base1=LSB of Input  bit0=0  base0=LSB of Input  dbl_ovrd=off  block_type=slice
  slice_sel_bottom_3 : xbsIndex_r4/Slice  nbits=1  boolean_output=off  mode=Lower Bit Location + Width  bit1=0  base1=LSB of Input  bit0=0  base0=LSB of Input  dbl_ovrd=off  block_type=slice
  slice_sel_top_{1..4} (4 alike) : xbsIndex_r4/Slice  nbits=1  boolean_output=on  mode=Upper Bit Location + Width  bit1=0  base1=MSB of Input  bit0=0  base0=MSB of Input  dbl_ovrd=off  block_type=slice
  sync_delay_fast : monroe_library/sync_delay_fast  SystemSampleTime=-1  delay_len=12
  coeff : Outport
  sel : Outport  Port=2
  sync_out : Outport  Port=3
  wires:
  sync/1 -> Counter/1, sync_delay_fast/1
  coeff_sync_late_3/1 -> coeff_sync_early_4/1, coeff_gen3/1(sync)
  coeff_sync_late_4/1 -> delay_sync_final/1, coeff_gen4/1(sync)
  sel_delay1/1 -> slice_sel_bottom_1/1, slice_sel_top_1/1
  sel_delay2/1 -> slice_sel_bottom_2/1, slice_sel_top_2/1
  sel_delay3/1 -> slice_sel_bottom_3/1, slice_sel_top_3/1
  delay_sync_final/1 -> sync_out/1
  concat/1 -> sel/1
  slice_sel_top_4/1 -> concat/4
  slice_sel_top_3/1 -> concat/3
  slice_sel_top_2/1 -> concat/2
  slice_sel_top_1/1 -> concat/1
  sel_delay4/1 -> slice_sel_top_4/1
  slice_sel_bottom_3/1 -> sel_delay4/1
  slice_sel_bottom_2/1 -> sel_delay3/1
  slice_sel_bottom_1/1 -> sel_delay2/1
  Counter/1 -> sel_delay1/1
  cram/1(out) -> coeff/1
  coeff_gen4/1(coeff) -> cram/2(in1)
  coeff_gen3/1(coeff) -> cram/1(in0)
  coeff_sync_early_4/1 -> coeff_sync_late_4/1
  coeff_sync_early_3/1 -> coeff_sync_late_3/1
  sync_delay_fast/1 -> coeff_sync_early_3/1

== system monroe_library/bit_reverse ==
  in : Inport
  Concat : xbsIndex_r4/Concat  num_inputs=5  dbl_ovrd=off  block_type=concat
  Slice : xbsIndex_r4/Slice  nbits=1  boolean_output=off  mode=Lower Bit Location + Width  bit1=0  base1=MSB of Input  bit0=0  base0=MSB of Input  dbl_ovrd=off  block_type=slice
  Slice1 : xbsIndex_r4/Slice  nbits=1  boolean_output=off  mode=Lower Bit Location + Width  bit1=1  base1=MSB of Input  bit0=0  base0=MSB of Input  dbl_ovrd=off  block_type=slice
  Slice2 : xbsIndex_r4/Slice  nbits=1  boolean_output=off  mode=Lower Bit Location + Width  bit1=2  base1=MSB of Input  bit0=0  base0=MSB of Input  dbl_ovrd=off  block_type=slice
  Slice3 : xbsIndex_r4/Slice  nbits=1  boolean_output=off  mode=Lower Bit Location + Width  bit1=3  base1=MSB of Input  bit0=0  base0=MSB of Input  dbl_ovrd=off  block_type=slice
  Slice4 : xbsIndex_r4/Slice  nbits=1  boolean_output=off  mode=Lower Bit Location + Width  bit1=4  base1=MSB of Input  bit0=0  base0=MSB of Input  dbl_ovrd=off  block_type=slice
  out : Outport
  wires:
  Slice/1 -> Concat/1
  Slice1/1 -> Concat/2
  Slice2/1 -> Concat/3
  Slice3/1 -> Concat/4
  Slice4/1 -> Concat/5
  Concat/1 -> out/1
  in/1 -> Slice/1, Slice1/1, Slice2/1, Slice3/1, Slice4/1

== system monroe_library/bulk_delay ==
  in1 : Inport
  in2 : Inport  Port=2
  in3 : Inport  Port=3
  in4 : Inport  Port=4
  in5 : Inport  Port=5
  in6 : Inport  Port=6
  in7 : Inport  Port=7
  in8 : Inport  Port=8
  in9 : Inport  Port=9
  delay_{1..9} (9 alike) : xbsIndex_r4/Delay  en=off  latency=5  dbl_ovrd=off  reg_retiming=off  block_type=delay
  out1 : Outport
  out2 : Outport  Port=2
  out3 : Outport  Port=3
  out4 : Outport  Port=4
  out5 : Outport  Port=5
  out6 : Outport  Port=6
  out7 : Outport  Port=7
  out8 : Outport  Port=8
  out9 : Outport  Port=9
  wires:
  delay_9/1 -> out9/1
  in9/1 -> delay_9/1
  delay_8/1 -> out8/1
  in8/1 -> delay_8/1
  delay_7/1 -> out7/1
  in7/1 -> delay_7/1
  delay_6/1 -> out6/1
  in6/1 -> delay_6/1
  delay_5/1 -> out5/1
  in5/1 -> delay_5/1
  delay_4/1 -> out4/1
  in4/1 -> delay_4/1
  delay_3/1 -> out3/1
  in3/1 -> delay_3/1
  delay_2/1 -> out2/1
  in2/1 -> delay_2/1
  delay_1/1 -> out1/1
  in1/1 -> delay_1/1

== system monroe_library/c_to_ri ==
  c : Inport
  force_im : xbsIndex_r4/Reinterpret  force_arith_type=on  arith_type="Signed  (2's comp)"  force_bin_pt=on  bin_pt=bin_pt  block_type=reinterpret
      settings: infoedit="Changes signal type without altering the binary representation.   You can changed the signal between signed and unsigned, and relocate the binary point.<P><P>Hardware notes: In hardware this block costs nothing.<P><P>Example:  Suppose the input is 6 bits wide, signed, with 2 fractional bits, and the output is forced to unsigned with 0 fractional bits.  Then an input of -2.0 (1110.00 in binary 2's complement) becomes an output of 56 (111000 in binary)."  block_version=9.1.01
  force_re : xbsIndex_r4/Reinterpret  force_arith_type=on  arith_type="Signed  (2's comp)"  force_bin_pt=on  bin_pt=bin_pt  block_type=reinterpret
      settings: infoedit="Changes signal type without altering the binary representation.   You can changed the signal between signed and unsigned, and relocate the binary point.<P><P>Hardware notes: In hardware this block costs nothing.<P><P>Example:  Suppose the input is 6 bits wide, signed, with 2 fractional bits, and the output is forced to unsigned with 0 fractional bits.  Then an input of -2.0 (1110.00 in binary 2's complement) becomes an output of 56 (111000 in binary)."  block_version=9.1.01
  slice_im : xbsIndex_r4/Slice  nbits=n_bits  boolean_output=off  mode=Lower Bit Location + Width  bit1=0  base1=MSB of Input  bit0=0  base0=LSB of Input  dbl_ovrd=off  block_type=slice
      settings: infoedit="Extracts a given range of bits from each input sample and presents it at the output.  The output type is ordinarily unsigned with binary point at zero, but can be Boolean when the slice is one bit wide.<P><P>Hardware notes: In hardware this block costs nothing."  block_version=9.1.01
  slice_re : xbsIndex_r4/Slice  nbits=n_bits  boolean_output=off  mode=Upper Bit Location + Width  bit1=0  base1=MSB of Input  bit0=0  base0=LSB of Input  dbl_ovrd=off  block_type=slice
      settings: infoedit="Extracts a given range of bits from each input sample and presents it at the output.  The output type is ordinarily unsigned with binary point at zero, but can be Boolean when the slice is one bit wide.<P><P>Hardware notes: In hardware this block costs nothing."  block_version=9.1.01
  re : Outport
  im : Outport  Port=2
  wires:
  c/1 -> slice_im/1, slice_re/1
  force_im/1 -> im/1
  force_re/1 -> re/1
  slice_im/1 -> force_im/1
  slice_re/1 -> force_re/1
